simulink model "Subsystem"  (R2024b)
settings: Solver=VariableStepAuto  StartTime=0.0  StopTime=10.0  RelTol=1e-3
InitFcn:
  | J =0.01;
  | b = 0.1;
  | K = 0.01;
  | R = 1;
  | kb =0.01;
  | L = 0.5;
  | Kp=550;
  | ki = 500;
  | Ts = 0.01;
  | Kd =0.01;
settings Model: Creator=chall  LastModifiedBy=Sagar
settings DataIOCC: SaveOutput=off  SaveTime=off

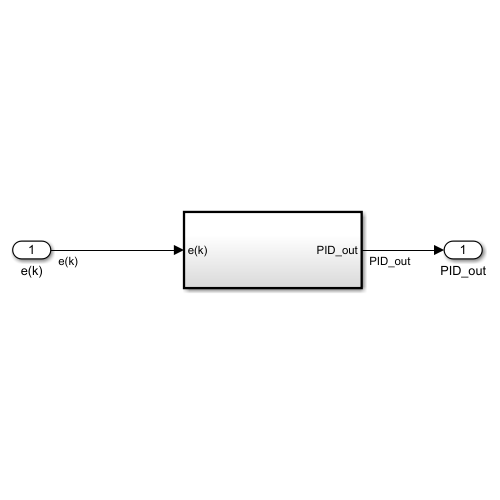
[thumbnail: Simulink's stored preview of the top-level diagram]
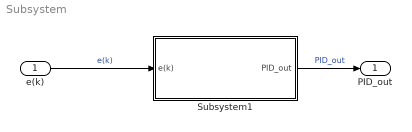
== system Subsystem ==
  e(k) : Inport  OutDataTypeStr=double  PortDimensions=1  SampleTime=0
  Subsystem1 : Subsystem  TreatAsAtomicUnit=on
  PID_out : Outport  OutDataTypeStr=double  PortDimensions=1  SampleTime=0
  wires:
  Subsystem1/1(PID_out) -> PID_out/1  "PID_out"
  e(k)/1 -> Subsystem1/1(e(k))  "e(k)"

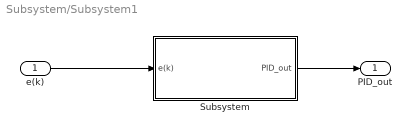
== system Subsystem/Subsystem1 ==
  e(k) : Inport
  Subsystem : Subsystem  TreatAsAtomicUnit=on
  PID_out : Outport
  wires:
  e(k)/1 -> Subsystem/1(e(k))
  Subsystem/1(PID_out) -> PID_out/1

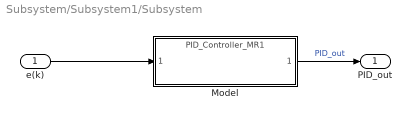
== system Subsystem/Subsystem1/Subsystem ==
  e(k) : Inport
  Model : ModelReference  ModelNameDialog=PID_Controller_MR1  SimulationMode=Normal  ModelReferenceVersion=1.4
  PID_out : Outport
  wires:
  e(k)/1 -> Model/1
  Model/1 -> PID_out/1  "PID_out"
